simulink model "Prova_slk"  (R2023b)
settings: Solver=VariableStepAuto  StartTime=0.0  StopTime=Tend_slk  FixedStep=0.002  RelTol=1e-3  EnableMultiTasking=on
values from neighbouring files (symbols this model uses):
  Alin = [0  1; 0  0]    [system_lin0_1dof_new_Ixx.mat]
  Blin = [0 18.1818181818]    [system_lin0_1dof_new_Ixx.mat]
  Kv = -9.438e-05    [K_pole_1dof_new_Ixx.mat]    (also in Prova.m = K(:,3))
  Kx = [0.0023705 0.0198]    [K_pole_1dof_new_Ixx.mat]    (also in Prova.m = K(:,1:2))
  param = [Ixx;Iyy;Izz;l;k1;k2;k3;k4;b;m]    [Nuovo_main_H2_1dof.m]    (also in Nuovo_main_pole_1dof.m; Prova.m)
  Ts_slk = 0.01    [Nuovo_main_H2_1dof.m]    (also in Nuovo_main_pole_1dof.m; Prova.m)
  x0 = [1;0]*0.01    [Nuovo_main_H2_1dof.m]    (also in Nuovo_main_pole_1dof.m; Prova.m = [0;0])
undefined symbols (not defined in the file or in its folder): Kd, Ki, Kp, x_eq
libraries: simulink x5, cstblocks x4, slpidlib x4
settings Model: ExtModeTrigDuration=10000  Creator=asus  LastModifiedBy=asus
settings SolverCC: AlgebraicLoopSolver=TrustRegion  PositivePriorityOrder=on  AutoInsertRateTranBlk=on
settings DataIOCC: ReturnWorkspaceOutputs=off
settings OptimizationCC: LifeSpan=inf
settings DebuggingCC: UnconnectedInputMsg=warning  UnconnectedOutputMsg=warning  UnconnectedLineMsg=warning  ArithmeticOperatorsInVariantConditions=warning
settings ModelReferenceCC: EnableRefExpFcnMdlSchedulingChecks=on
settings SFSimCC: SimUseLocalCustomCode=off  CustomCodeUndefinedFunction=UseInterfaceOnly
settings RTWCC: Description=QUARC Win64 Target  SystemTargetFile=quarc_win64.tlc  TemplateMakefile=quarc_default_tmf  RTWUseLocalCustomCode=off
settings CodeAppCC: StateflowObjectComments=on
settings STFCustomTargetCC: TargetPreCompLibLocation=C:\PROGRA~3\QUARC\lib\2016a\win64\release  ConcurrentExecutionCompliant=on  GRTInterface=on  SystemTargetFile=quarc_win64.tlc
settings GRTTargetCC: TargetPreCompLibLocation=C:\PROGRA~3\QUARC\lib\2016a\win64\release  ParMdlRefBuildCompliant=off  CompOptLevelCompliant=off  CombineOutputUpdateFcns=off  MatFileLogging=off  CPPClassGenCompliant=off  GRTInterface=on  UseToolchainInfoCompliant=off  ExtMode=on  ExtModeMexFile=quarc_comm
settings ConfigComp: CovMetricSettings=dswe

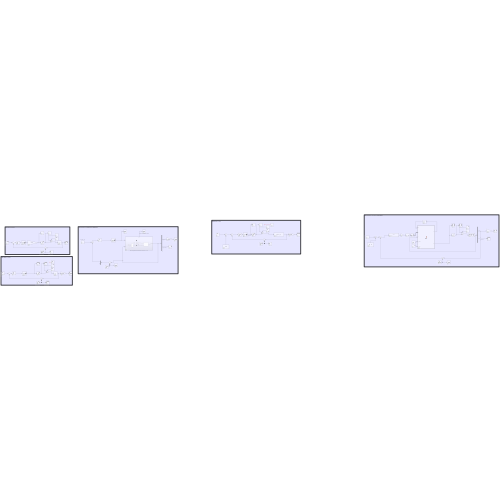
[thumbnail: Simulink's stored preview of the top-level diagram]
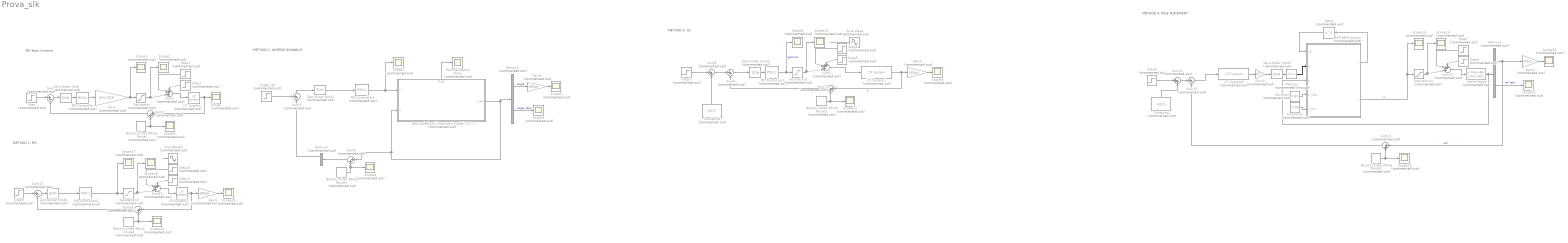
== system Prova_slk ==
  note: METHOD 3: H2
  note: METHOD 2: INVERSE DYNAMICS
  note: PID fatto insieme
  note: METHOD 4: POLE PLACEMENT
  note: METHOD 1: PID
  Band-Limited White Noise{,1..4} (5 alike) : simulink/Sources/Band-Limited White Noise  Commented=on  Cov=[0.0001]  Ts=0.05  seed=[23341]
  Constant : Constant  Commented=on  Value=0.85  SampleTime=Ts_slk
  Constant1 : Constant  Commented=on  Value=x0(1)
  Constant2 : Constant  Commented=on  Value=-0.85  SampleTime=Ts_slk
  Constant4 : Constant  Commented=on  Value=x0(1)
  Decoupled and linearized model: 1/s^2 : Subsystem  Commented=on
      settings: PortSchema="{\"entries\":[{\"content\":{\"sides\":[{\"content\":{\"connectorIds\":[\"In1\",\"In2\"]},\"type\":\"ConnectorPlacement.EquallySpacedRectSide\",\"uuid\":\"00f00ec3-2aa5-4d08-af17-15441a555b9c\"},{\"content\":{\"connectorIds\":[\"Out1\"],\"side\":\"RIGHT\"},\"type\":\"ConnectorPlacement.EquallySpacedRectSide\",\"uuid\":\"964782b2-5db9-4cc7-bfcc-68e482a20668\"},{\"content\":{\"connectorIds\":[\"Out2\"],\"side\":\"TOP\"},\"type\":\"ConnectorPlacement.EquallySpacedRectSide\",\"uuid\":\"d9fa26a1-22f0-4c54-8a50-c97da7d25523\"}]},\"type\":\"ConnectorPlacement.EquallySpacedConnector\",\"uuid\":\"aed33859-7045-4c34-9a7e-a67dc13ff2cc\"}],\"packageUris\":[\"http://schema.mathworks.com/mf0/Connector/R2020b\"],\"version\":\"1.0\"}"
  Delay : Delay  Commented=on  DelayLength=1  SampleTime=Ts_slk
  Demux1 : Demux  Commented=on  Outputs=2
  Demux2 : Demux  Commented=on  Outputs=2
  Demux3 : Demux  Commented=on  Outputs=2
  Gain : Gain  Commented=on  Gain=5*0.055
  Gain{1..2,4..5} (4 alike) : Gain  Commented=on  Gain=180/pi
  Gain3 : Gain  Commented=on  Gain=35
  LTI System : cstblocks/LTI System  Commented=on  sys=G  IC=[]  PadeOrder=0
  LTI System1 : cstblocks/LTI System  Commented=on  sys=stable_sys  IC=[]  PadeOrder=0
  LTI System2 : cstblocks/LTI System  Commented=on  sys=G  IC=[]  PadeOrder=0
  LTI System6 : cstblocks/LTI System  Commented=on  sys=filter_d  IC=[]  PadeOrder=0
  MATLAB Function : MATLAB Function  Commented=on  TreatAsAtomicUnit=on
  Memory : Memory  Commented=through
  PID Controller : slpidlib/PID Controller  Commented=on  Controller=PID  Form=Parallel  TimeDomain=Continuous-time  UseExternalTs=off  SampleTime=Ts_slk  IntegratorMethod=Forward Euler  FilterMethod=Forward Euler  ControllerParametersSource=internal  P=0.2  I=0.01  UseKiTs=off  D=1  N=10  UseFilter=on  TunerSelectOption=Transfer Function Based (PID Tuner App)  InitialConditionSource=internal  InitialConditionForIntegrator=0  InitialConditionForFilter=0  DifferentiatorICPrevScaledInput=0  ExternalReset=none  TrackingMode=off  Kt=1  LimitOutput=on  SatLimitsSource=internal  UpperSaturationLimit=1.2  LowerSaturationLimit=-1.2  LinearizeAsGain=on  AntiWindupMode=clamping  Kb=1  LimitIntegrator=off  UpperIntegratorSaturationLimit=inf  LowerIntegratorSaturationLimit=-inf  POutMin=[]  POutMax=[]  IOutMin=[]  IOutMax=[]  DOutMin=[]  DOutMax=[]  NOutMin=[]  NOutMax=[]  SumOutMin=[]  SumOutMax=[]  SaturationOutMin=[]  SaturationOutMax=[]  PParamMin=[]  PParamMax=[]  IParamMin=[]  IParamMax=[]  DParamMin=[]  DParamMax=[]  NParamMin=[]  NParamMax=[]  KbParamMin=[]  KbParamMax=[]  KtParamMin=[]  KtParamMax=[]  KbOutMin=[]  KbOutMax=[]  KtOutMin=[]  KtOutMax=[]  IntegratorOutMin=[]  IntegratorOutMax=[]  FilterOutMin=[]  FilterOutMax=[]  SumI1OutMin=[]  SumI1OutMax=[]  SumI2OutMin=[]  SumI2OutMax=[]  SumI3OutMin=[]  SumI3OutMax=[]  SumI4OutMin=[]  SumI4OutMax=[]  SumDOutMin=[]  SumDOutMax=[]  DifferentiatorOutMin=[]  DifferentiatorOutMax=[]  FilterDiffOutCoefMin=[]  FilterDiffOutCoefMax=[]  ReciprocalOutMin=[]  ReciprocalOutMax=[]  SumDenOutMin=[]  SumDenOutMax=[]  SumNumOutMin=[]  SumNumOutMax=[]  DivideOutMin=[]  DivideOutMax=[]  UdiffTsProdOutMin=[]  UdiffTsProdOutMax=[]  NTsProdOutMin=[]  NTsProdOutMax=[]  UintegralTsProdOutMin=[]  UintegralTsProdOutMax=[]  UngainTsProdOutMin=[]  UngainTsProdOutMax=[]  ClampingZeroOutDataTypeStr=Inherit: Inherit via back propagation  ClampingZeroOutMin=[]  ClampingZeroOutMax=[]  FilterDenConstantOutDataTypeStr=Inherit: Inherit via back propagation  FilterDenConstantOutMin=[]  FilterDenConstantOutMax=[]  PCopyOutDataTypeStr=Inherit: Inherit via back propagation  PCopyOutMin=[]  PCopyOutMax=[]  NCopyOutDataTypeStr=Inherit: Inherit via back propagation  NCopyOutMin=[]  NCopyOutMax=[]  IntegratorContinuousStateAttributes=''  IntegratorStateMustResolveToSignalObject=off  IntegratorRTWStateStorageClass=Auto  FilterContinuousStateAttributes=''  FilterStateMustResolveToSignalObject=off  FilterRTWStateStorageClass=Auto  ParallelPVariant=InternalParameters  IdealPVariant=Disabled  IVariant=InternalParameters  DVariant=InternalParameters  IntegratorVariant=Continuous  SatVariant=Enabled  AWVariant=ContClampingParallel  PCopyVariant=Disabled  TRVariant=Disabled  FdbkBlocksVariant=Forward  IdealPFdbkVariant=Disabled  SatFdbkVariant=Disabled  DerivativeFilterVariant=ContFilter  NVariant=InternalParameters  NCopyVariant=Disabled  FilterICVariant=InternalICsFilter  IntegratorICVariant=InternalICs  ExternalResetVariant=Disabled  TRSumVariant=Passthrough  SumFdbkVariant=Disabled  SumVariant=Sum_PID  TsampFilterVariant=InternalTs  TsampNgainVariant=Passthrough  TsampIntegralVariant=Disabled_SignalSpec  ExternalSaturationOutDataTypeStr=Inherit: Same as second input
  PID Controller1 : slpidlib/PID Controller  Commented=on  Controller=PID  Form=Parallel  TimeDomain=Discrete-time  UseExternalTs=off  SampleTime=Ts_slk  IntegratorMethod=Forward Euler  FilterMethod=Forward Euler  ControllerParametersSource=internal  P=Kp  I=Ki  UseKiTs=off  D=Kd  N=4.862432089028  UseFilter=on  TunerSelectOption=Transfer Function Based (PID Tuner App)  InitialConditionSource=internal  InitialConditionForIntegrator=0  InitialConditionForFilter=0  DifferentiatorICPrevScaledInput=0  ExternalReset=none  TrackingMode=off  Kt=1  LimitOutput=on  SatLimitsSource=internal  UpperSaturationLimit=1.2  LowerSaturationLimit=-1.2  LinearizeAsGain=on  AntiWindupMode=clamping  Kb=1  LimitIntegrator=off  UpperIntegratorSaturationLimit=inf  LowerIntegratorSaturationLimit=-inf  POutMin=[]  POutMax=[]  IOutMin=[]  IOutMax=[]  DOutMin=[]  DOutMax=[]  NOutMin=[]  NOutMax=[]  SumOutMin=[]  SumOutMax=[]  SaturationOutMin=[]  SaturationOutMax=[]  PParamMin=[]  PParamMax=[]  IParamMin=[]  IParamMax=[]  DParamMin=[]  DParamMax=[]  NParamMin=[]  NParamMax=[]  KbParamMin=[]  KbParamMax=[]  KtParamMin=[]  KtParamMax=[]  KbOutMin=[]  KbOutMax=[]  KtOutMin=[]  KtOutMax=[]  IntegratorOutMin=[]  IntegratorOutMax=[]  FilterOutMin=[]  FilterOutMax=[]  SumI1OutMin=[]  SumI1OutMax=[]  SumI2OutMin=[]  SumI2OutMax=[]  SumI3OutMin=[]  SumI3OutMax=[]  SumI4OutMin=[]  SumI4OutMax=[]  SumDOutMin=[]  SumDOutMax=[]  DifferentiatorOutMin=[]  DifferentiatorOutMax=[]  FilterDiffOutCoefMin=[]  FilterDiffOutCoefMax=[]  ReciprocalOutMin=[]  ReciprocalOutMax=[]  SumDenOutMin=[]  SumDenOutMax=[]  SumNumOutMin=[]  SumNumOutMax=[]  DivideOutMin=[]  DivideOutMax=[]  UdiffTsProdOutMin=[]  UdiffTsProdOutMax=[]  NTsProdOutMin=[]  NTsProdOutMax=[]  UintegralTsProdOutMin=[]  UintegralTsProdOutMax=[]  UngainTsProdOutMin=[]  UngainTsProdOutMax=[]  ClampingZeroOutDataTypeStr=Inherit: Inherit via back propagation  ClampingZeroOutMin=[]  ClampingZeroOutMax=[]  FilterDenConstantOutDataTypeStr=Inherit: Inherit via back propagation  FilterDenConstantOutMin=[]  FilterDenConstantOutMax=[]  PCopyOutDataTypeStr=Inherit: Inherit via back propagation  PCopyOutMin=[]  PCopyOutMax=[]  NCopyOutDataTypeStr=Inherit: Inherit via back propagation  NCopyOutMin=[]  NCopyOutMax=[]  IntegratorContinuousStateAttributes=''  IntegratorStateMustResolveToSignalObject=off  IntegratorRTWStateStorageClass=Auto  FilterContinuousStateAttributes=''  FilterStateMustResolveToSignalObject=off  FilterRTWStateStorageClass=Auto  ParallelPVariant=InternalParameters  IdealPVariant=Disabled  IVariant=InternalParameters  DVariant=InternalParameters  IntegratorVariant=Discrete  SatVariant=Enabled  AWVariant=DiscClampingParallel  PCopyVariant=Disabled  TRVariant=Disabled  FdbkBlocksVariant=Forward  IdealPFdbkVariant=Disabled  SatFdbkVariant=Disabled  DerivativeFilterVariant=ForwardEulerFilter  NVariant=InternalParameters  NCopyVariant=Disabled  FilterICVariant=InternalICsFilter  IntegratorICVariant=InternalICs  ExternalResetVariant=Disabled  TRSumVariant=Passthrough  SumFdbkVariant=Disabled  SumVariant=Sum_PID  TsampFilterVariant=InternalTs  TsampNgainVariant=Passthrough  TsampIntegralVariant=Disabled_SignalSpec  ExternalSaturationOutDataTypeStr=Inherit: Same as second input
  PID Controller2 : slpidlib/PID Controller  Commented=on  Controller=PID  Form=Parallel  TimeDomain=Discrete-time  UseExternalTs=off  SampleTime=Ts_slk  IntegratorMethod=Forward Euler  FilterMethod=Forward Euler  ControllerParametersSource=internal  P=0.180109037198918  I=0.150719618455462  UseKiTs=off  D=0.0291322547663788  N=114.28279760416  UseFilter=on  TunerSelectOption=Transfer Function Based (PID Tuner App)  InitialConditionSource=internal  InitialConditionForIntegrator=0  InitialConditionForFilter=0  DifferentiatorICPrevScaledInput=0  ExternalReset=none  TrackingMode=off  Kt=1  LimitOutput=on  SatLimitsSource=internal  UpperSaturationLimit=1.2  LowerSaturationLimit=-1.2  LinearizeAsGain=on  AntiWindupMode=clamping  Kb=1  LimitIntegrator=off  UpperIntegratorSaturationLimit=inf  LowerIntegratorSaturationLimit=-inf  POutMin=[]  POutMax=[]  IOutMin=[]  IOutMax=[]  DOutMin=[]  DOutMax=[]  NOutMin=[]  NOutMax=[]  SumOutMin=[]  SumOutMax=[]  SaturationOutMin=[]  SaturationOutMax=[]  PParamMin=[]  PParamMax=[]  IParamMin=[]  IParamMax=[]  DParamMin=[]  DParamMax=[]  NParamMin=[]  NParamMax=[]  KbParamMin=[]  KbParamMax=[]  KtParamMin=[]  KtParamMax=[]  KbOutMin=[]  KbOutMax=[]  KtOutMin=[]  KtOutMax=[]  IntegratorOutMin=[]  IntegratorOutMax=[]  FilterOutMin=[]  FilterOutMax=[]  SumI1OutMin=[]  SumI1OutMax=[]  SumI2OutMin=[]  SumI2OutMax=[]  SumI3OutMin=[]  SumI3OutMax=[]  SumI4OutMin=[]  SumI4OutMax=[]  SumDOutMin=[]  SumDOutMax=[]  DifferentiatorOutMin=[]  DifferentiatorOutMax=[]  FilterDiffOutCoefMin=[]  FilterDiffOutCoefMax=[]  ReciprocalOutMin=[]  ReciprocalOutMax=[]  SumDenOutMin=[]  SumDenOutMax=[]  SumNumOutMin=[]  SumNumOutMax=[]  DivideOutMin=[]  DivideOutMax=[]  UdiffTsProdOutMin=[]  UdiffTsProdOutMax=[]  NTsProdOutMin=[]  NTsProdOutMax=[]  UintegralTsProdOutMin=[]  UintegralTsProdOutMax=[]  UngainTsProdOutMin=[]  UngainTsProdOutMax=[]  ClampingZeroOutDataTypeStr=Inherit: Inherit via back propagation  ClampingZeroOutMin=[]  ClampingZeroOutMax=[]  FilterDenConstantOutDataTypeStr=Inherit: Inherit via back propagation  FilterDenConstantOutMin=[]  FilterDenConstantOutMax=[]  PCopyOutDataTypeStr=Inherit: Inherit via back propagation  PCopyOutMin=[]  PCopyOutMax=[]  NCopyOutDataTypeStr=Inherit: Inherit via back propagation  NCopyOutMin=[]  NCopyOutMax=[]  IntegratorContinuousStateAttributes=''  IntegratorStateMustResolveToSignalObject=off  IntegratorRTWStateStorageClass=Auto  FilterContinuousStateAttributes=''  FilterStateMustResolveToSignalObject=off  FilterRTWStateStorageClass=Auto  ParallelPVariant=InternalParameters  IdealPVariant=Disabled  IVariant=InternalParameters  DVariant=InternalParameters  IntegratorVariant=Discrete  SatVariant=Enabled  AWVariant=DiscClampingParallel  PCopyVariant=Disabled  TRVariant=Disabled  FdbkBlocksVariant=Forward  IdealPFdbkVariant=Disabled  SatFdbkVariant=Disabled  DerivativeFilterVariant=ForwardEulerFilter  NVariant=InternalParameters  NCopyVariant=Disabled  FilterICVariant=InternalICsFilter  IntegratorICVariant=InternalICs  ExternalResetVariant=Disabled  TRSumVariant=Passthrough  SumFdbkVariant=Disabled  SumVariant=Sum_PID  TsampFilterVariant=InternalTs  TsampNgainVariant=Passthrough  TsampIntegralVariant=Disabled_SignalSpec  ExternalSaturationOutDataTypeStr=Inherit: Same as second input
  PID Controller3 : slpidlib/PID Controller  Commented=on  Controller=PID  Form=Parallel  TimeDomain=Discrete-time  UseExternalTs=off  SampleTime=Ts_slk  IntegratorMethod=Forward Euler  FilterMethod=Forward Euler  ControllerParametersSource=internal  P=0.0408494379196507*4  I=0.00382471475812365  UseKiTs=off  D=0.107131307975801  N=10.9079405084324  UseFilter=on  TunerSelectOption=Transfer Function Based (PID Tuner App)  InitialConditionSource=internal  InitialConditionForIntegrator=0  InitialConditionForFilter=0  DifferentiatorICPrevScaledInput=0  ExternalReset=none  TrackingMode=off  Kt=1  LimitOutput=on  SatLimitsSource=internal  UpperSaturationLimit=1.2  LowerSaturationLimit=-1.2  LinearizeAsGain=on  AntiWindupMode=clamping  Kb=1  LimitIntegrator=off  UpperIntegratorSaturationLimit=inf  LowerIntegratorSaturationLimit=-inf  POutMin=[]  POutMax=[]  IOutMin=[]  IOutMax=[]  DOutMin=[]  DOutMax=[]  NOutMin=[]  NOutMax=[]  SumOutMin=[]  SumOutMax=[]  SaturationOutMin=[]  SaturationOutMax=[]  PParamMin=[]  PParamMax=[]  IParamMin=[]  IParamMax=[]  DParamMin=[]  DParamMax=[]  NParamMin=[]  NParamMax=[]  KbParamMin=[]  KbParamMax=[]  KtParamMin=[]  KtParamMax=[]  KbOutMin=[]  KbOutMax=[]  KtOutMin=[]  KtOutMax=[]  IntegratorOutMin=[]  IntegratorOutMax=[]  FilterOutMin=[]  FilterOutMax=[]  SumI1OutMin=[]  SumI1OutMax=[]  SumI2OutMin=[]  SumI2OutMax=[]  SumI3OutMin=[]  SumI3OutMax=[]  SumI4OutMin=[]  SumI4OutMax=[]  SumDOutMin=[]  SumDOutMax=[]  DifferentiatorOutMin=[]  DifferentiatorOutMax=[]  FilterDiffOutCoefMin=[]  FilterDiffOutCoefMax=[]  ReciprocalOutMin=[]  ReciprocalOutMax=[]  SumDenOutMin=[]  SumDenOutMax=[]  SumNumOutMin=[]  SumNumOutMax=[]  DivideOutMin=[]  DivideOutMax=[]  UdiffTsProdOutMin=[]  UdiffTsProdOutMax=[]  NTsProdOutMin=[]  NTsProdOutMax=[]  UintegralTsProdOutMin=[]  UintegralTsProdOutMax=[]  UngainTsProdOutMin=[]  UngainTsProdOutMax=[]  ClampingZeroOutDataTypeStr=Inherit: Inherit via back propagation  ClampingZeroOutMin=[]  ClampingZeroOutMax=[]  FilterDenConstantOutDataTypeStr=Inherit: Inherit via back propagation  FilterDenConstantOutMin=[]  FilterDenConstantOutMax=[]  PCopyOutDataTypeStr=Inherit: Inherit via back propagation  PCopyOutMin=[]  PCopyOutMax=[]  NCopyOutDataTypeStr=Inherit: Inherit via back propagation  NCopyOutMin=[]  NCopyOutMax=[]  IntegratorContinuousStateAttributes=''  IntegratorStateMustResolveToSignalObject=off  IntegratorRTWStateStorageClass=Auto  FilterContinuousStateAttributes=''  FilterStateMustResolveToSignalObject=off  FilterRTWStateStorageClass=Auto  ParallelPVariant=InternalParameters  IdealPVariant=Disabled  IVariant=InternalParameters  DVariant=InternalParameters  IntegratorVariant=Discrete  SatVariant=Enabled  AWVariant=DiscClampingParallel  PCopyVariant=Disabled  TRVariant=Disabled  FdbkBlocksVariant=Forward  IdealPFdbkVariant=Disabled  SatFdbkVariant=Disabled  DerivativeFilterVariant=ForwardEulerFilter  NVariant=InternalParameters  NCopyVariant=Disabled  FilterICVariant=InternalICsFilter  IntegratorICVariant=InternalICs  ExternalResetVariant=Disabled  TRSumVariant=Passthrough  SumFdbkVariant=Disabled  SumVariant=Sum_PID  TsampFilterVariant=InternalTs  TsampNgainVariant=Passthrough  TsampIntegralVariant=Disabled_SignalSpec  ExternalSaturationOutDataTypeStr=Inherit: Same as second input
  Post saturation block : Scope  Commented=on
  Saturation : Saturate  Commented=on  UpperLimit=1.2  LowerLimit=-1.2
  Saturation1 : Saturate  Commented=on  UpperLimit=1.2  LowerLimit=-1.2
  Saturation2 : Saturate  Commented=on  UpperLimit=0.85  LowerLimit=-0.85
  Saturation3 : Saturate  Commented=on  UpperLimit=1.2  LowerLimit=-1.2
  Scope{,1..20} (21 alike) : Scope  Commented=on
  Sine Wave : Sin  Commented=on  Amplitude=0.2  Frequency=4  SampleTime=Ts_slk
  Sine Wave2 : Sin  Commented=on  Amplitude=0.2  Frequency=5  SampleTime=Ts_slk
  State-Space : StateSpace  Commented=on  A=Alin  B=Blin  C=eye(2)  D=[0;0]  InitialCondition=0
  Step : Step  Commented=on  Time=0  After=0.5  SampleTime=Ts_slk
  Step{1,4,7,10} (4 alike) : Step  Commented=on  Time=100  After=0.2  SampleTime=Ts_slk
  Step{2,5,8,11} (4 alike) : Step  Commented=on  Time=100.1  After=-0.2  SampleTime=Ts_slk
  Step3 : Step  Commented=on  Time=80  Before=0.52  After=0  SampleTime=Ts_slk
  Step6 : Step  Commented=on  Time=0  After=30*pi/180  SampleTime=Ts_slk
  Step9 : Step  Commented=on  Time=80  Before=0.5  After=0  SampleTime=Ts_slk
  Sum{,6,10,14} (4 alike) : Sum  Commented=on  Inputs=|+-
  Sum{1,5,12,15} (4 alike) : Sum  Commented=on  Inputs=+++|
  Sum{2,4,7,9,11,13,16} (7 alike) : Sum  Commented=on  Inputs=|++
  Sum3 : Sum  Commented=on  Inputs=+-|
  Zero-Order Hold{,1..4} (5 alike) : ZeroOrderHold  Commented=on  SampleTime=Ts_slk
  angle_ref : Step  Commented=on  Time=80  Before=30*pi/180  After=0  SampleTime=Ts_slk
  wires:
  Sum/1 -> Zero-Order Hold/1
  PID Controller/1 -> Gain/1
  Saturation/1 -> Scope2/1, Sum1/3
  Step/1 -> Sum/1
  Sum1/1 -> LTI System/1
  Step1/1 -> Sum1/2
  Step2/1 -> Sum1/1
  Zero-Order Hold/1 -> PID Controller/1
  LTI System/1 -> Sum2/1, Scope/1
  Band-Limited White Noise/1 -> Scope3/1, Sum2/2
  Gain/1 -> Saturation/1, Scope1/1
  Demux1/1 -> Gain4/1  "angle"
  Demux1/2 -> Scope6/1  "angle rate"
  Demux2/1 -> Sum3/2
  Sum3/1 -> Zero-Order Hold1/1
  angle_ref/1 -> Sum3/1
  PID Controller1/1 -> Scope7/1, Decoupled and linearized model: 1/s^2/1(v)
  Zero-Order Hold1/1 -> PID Controller1/1
  Band-Limited White Noise1/1 -> Scope4/1, Sum4/2
  Decoupled and linearized model: 1/s^2/2(Out1) -> Post saturation block/1
  Decoupled and linearized model: 1/s^2/1(x_out) -> Demux1/1, Sum4/1, Decoupled and linearized model: 1/s^2/2(x)
  Sum4/1 -> Demux2/1
  Step3/1 -> Sum9/1
  PID Controller2/1 -> Saturation1/1, Scope9/1  "gamma"
  Sum9/1 -> Sum6/1
  Constant4/1 -> Sum9/2
  LTI System1/1 -> Sum7/1, Gain5/1  "y"
  Zero-Order Hold2/1 -> PID Controller2/1
  Sum6/1 -> Zero-Order Hold2/1
  Saturation1/1 -> Scope10/1, Sum5/3
  Step5/1 -> Sum5/1
  Step4/1 -> Sum5/2
  Sum5/1 -> LTI System1/1
  Band-Limited White Noise2/1 -> Scope11/1, Sum7/2
  Sum7/1 -> Sum6/2
  Sine Wave/1 -> ?
  Step6/1 -> Sum11/1
  Constant1/1 -> Sum11/2
  Sum11/1 -> Sum10/1
  Sum13/1 -> Sum10/2
  Band-Limited White Noise3/1 -> Sum13/2, Scope15/1
  Zero-Order Hold4/1 -> PID Controller3/1
  Step10/1 -> Sum15/2
  Sum14/1 -> Zero-Order Hold4/1
  Band-Limited White Noise4/1 -> Scope19/1, Sum16/2
  Step11/1 -> Sum15/1
  Sum16/1 -> Sum14/2
  LTI System2/1 -> Sum16/1, Gain1/1
  Sum15/1 -> LTI System2/1
  Saturation3/1 -> Scope18/1, Sum15/3
  Step9/1 -> Sum14/1
  PID Controller3/1 -> Saturation3/1, Scope17/1
  Sine Wave2/1 -> ?
  Sum2/1 -> Sum/2
  Gain1/1 -> Scope16/1
  Gain4/1 -> Scope5/1
  Gain5/1 -> Scope8/1
  Gain2/1 -> Scope20/1
  Demux3/2 -> Scope12/1  "roll rate"
  Demux3/1 -> Gain2/1, Sum13/1  "roll"
  Sum10/1 -> LTI System6/1
  Gain3/1 -> Zero-Order Hold3/1
  MATLAB Function/1(v) -> Delay/1
  Constant2/1 -> MATLAB Function/5(u_min)
  Memory/1 -> MATLAB Function/2(e)
  MATLAB Function/2(u) -> Scope13/1, Saturation2/1  "u"
  State-Space/1 -> MATLAB Function/3(x), Demux3/1
  Zero-Order Hold3/1 -> Memory/1
  Saturation2/1 -> Scope14/1, Sum12/3
  Step8/1 -> Sum12/1
  Delay/1 -> MATLAB Function/1(v1)
  LTI System6/1 -> Gain3/1
  Constant/1 -> MATLAB Function/4(u_max)
  Sum12/1 -> State-Space/1
  Step7/1 -> Sum12/2

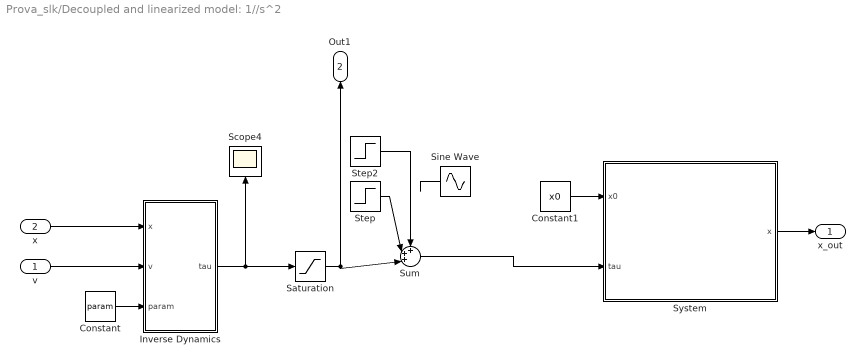
== system Prova_slk/Decoupled and linearized model: 1//s^2 ==
  v : Inport
  x : Inport  Port=2
  Constant : Constant  Value=param
  Constant1 : Constant  Value=x0
  Inverse Dynamics : MATLAB Function  TreatAsAtomicUnit=on
  Saturation : Saturate  UpperLimit=1.2  LowerLimit=-1.2
  Scope4 : Scope
  Sine Wave : Sin  Amplitude=0.2  Frequency=12  SampleTime=Ts_slk
  Step : Step  Time=100  After=0.2  SampleTime=Ts_slk
  Step2 : Step  Time=100.1  After=-0.2  SampleTime=Ts_slk
  Sum : Sum  Inputs=+++|
  System : Subsystem
  x_out : Outport
  Out1 : Outport  Port=2
  wires:
  x/1 -> Inverse Dynamics/1(x)
  Constant1/1 -> System/1(x0)
  v/1 -> Inverse Dynamics/2(v)
  Inverse Dynamics/1(tau) -> Saturation/1, Scope4/1
  Constant/1 -> Inverse Dynamics/3(param)
  System/1(x) -> x_out/1
  Sum/1 -> System/2("tau ")
  Step2/1 -> Sum/1
  Step/1 -> Sum/2
  Saturation/1 -> Out1/1, Sum/3
  Sine Wave/1 -> ?

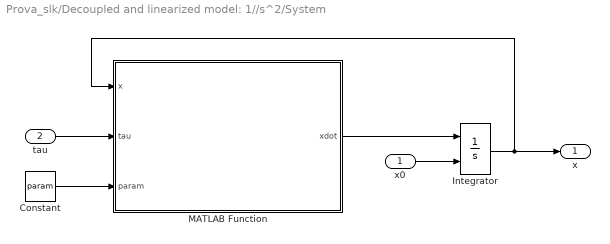
== system Prova_slk/Decoupled and linearized model: 1//s^2/System ==
  x0 : Inport
  "tau " : Inport  Port=2
  Constant : Constant  Value=param
  Integrator : Integrator  InitialConditionSource=external  InitialCondition=x_eq
  MATLAB Function : MATLAB Function  TreatAsAtomicUnit=on
  x : Outport
  wires:
  Integrator/1 -> MATLAB Function/1(x), x/1
  MATLAB Function/1(xdot) -> Integrator/1
  "tau "/1 -> MATLAB Function/2(tau)
  Constant/1 -> MATLAB Function/3(param)
  x0/1 -> Integrator/2

== matlab function Prova_slk/Decoupled and linearized model: 1//s^2/Inverse Dynamics ==
  data: x input; v input; tau output; param input
function tau = fcn(x,v,param)
% Inputs:
%           x       (model state)
%           v       (new input to the feedback system)           
%           param   (model parameters)
%
% Outputs:  tau  (torque)

% Parameters
g        =       9.81;           %  gravity acceleration (m/s^2)
Ixx      =       param(1,1);     %  moment of inertia 

% States
phi         =       x(1,1);      %  roll angle (rad)
phi_dot     =       x(2,1);      %  roll rate (rad/s)


cph         =       cos(phi);
sph         =       sin(phi);


% Inertia matrix
J= Ixx;

% control law
tau = 0;
tau = J*v;

== matlab function Prova_slk/Decoupled and linearized model: 1//s^2/System/MATLAB Function ==
  data: x input; tau input; xdot output; param input
function xdot=quadcopter(x,tau,param)
% Inputs:
%           x       (model state)
%           tau     (torque)           
%           param   (model parameters)
%
% Outputs:  x_dot  (derivative of the state with respect to time)

% Parameters
g        =       9.81;           %  gravity acceleration (m/s^2)
Ixx      =       param(1,1);     %  moment of inertia 

% States
phi         =       x(1,1);      %  roll angle (rad)
phi_dot     =       x(2,1);      %  roll rate (rad/s)


cph         =       cos(phi);
sph         =       sin(phi);

% State space model
xdot        = zeros(2,1);
xdot(1,1)   = phi_dot;
xdot(2,1)   = tau/Ixx;

== matlab function Prova_slk/MATLAB Function ==
  data: v output; v1 input; u output; e input; x input; u_max input; u_min input; Ts_slk parameter; Kx parameter; Kv parameter
function [v,u]  = fcn(v1,e,x,u_max,u_min,Ts_slk,Kx,Kv)
v   =   v1 + Ts_slk*e;
u   =  -Kv*v-Kx*x;
u   =   max(u_min,min(u_max,u));
v1  =   (-u-Kx*x)/Kv;
